simulink model "part2"  (R2025b)
settings: Solver=FixedStepAuto  StartTime=0.0  StopTime=t_end  FixedStep=h  RelTol=1e-3
values from neighbouring files (symbols this model uses):
  alpha = wind_coeff(:,1)*pi/180    [windCoefficients.m]
  Aw = [zeros(3,3), eye(3) ... (first row only)    [cal_jacobian.m]    (also in init.m = [zeros(3) eye(3))
  C_pitch = wind_coeff(:,6)    [windCoefficients.m]
  C_roll = wind_coeff(:,5)    [windCoefficients.m]
  C_yaw = wind_coeff(:,7)    [windCoefficients.m]
  Cw = [zeros(3) eye(3)]    [init.m]
  Cx = wind_coeff(:,2)    [windCoefficients.m]
  Cy = wind_coeff(:,3)    [windCoefficients.m]
  Cz = wind_coeff(:,4)    [windCoefficients.m]
  D = -[Xu  0   0 ... (first row only)    [ai_lqr.m]    (also in cal_jacobian.m = diag([d11, d22, d33]); compute_dp_gain_schedule.m = [2.6486e5       0           0; compute_integral_dp_gain_schedule.m = [2.6486e5       0           0; dp_lqSetPointTrack.m = [2.6486e5       0           0)
  K1 = [k11 0 0 ... (first row only)    [init.m]
  K2 = [k2 0 0 ... (first row only)    [init.m]
  K3 = [7.0184e6*0.1      0              0 ... (first row only)    [init.m]
  K4 = [7.0184e6*100      0              0 ... (first row only)    [init.m]
  Kp = M*Omega_n^2    [init_pid.m]
  M_inv = inv(M)    [cal_jacobian.m]    (also in init.m = M\eye(3))
  mu = 0.001    [SimulationParam.m]
  mu_w = 0.001    [init.m]
  psi_max = psi_wind_0 + deg2rad(5)    [init.m]
  psi_min = psi_wind_0 - deg2rad(5)    [init.m]
  psi_wind_0 = deg2rad(180)    [init.m]
  T_inv = T_mat\eye(3)    [init.m]
  U_bar = 10    [SimulationParam.m]    (also in init.m)
  Vc = -0.2    [SimulationParam.m]
  vessel = computeManeuveringModel(vessel, omega_p, plotFlag)    [init_pid.m]
undefined symbols (not defined in the file or in its folder): currentMode, DiscIntNeverNeededParam, Hoerner, Kd, Ki, thrusters
libraries: marine_gnc x2, marine_hydro x2, simulink x2
settings Model: Creator=jonbjor  LastModifiedBy=porpl
settings SolverCC: AlgebraicLoopSolver=TrustRegion
settings DataIOCC: ReturnWorkspaceOutputs=off
settings DebuggingCC: UnconnectedInputMsg=warning  UnconnectedOutputMsg=warning  UnconnectedLineMsg=warning  ArithmeticOperatorsInVariantConditions=warning
settings ModelReferenceCC: EnableRefExpFcnMdlSchedulingChecks=on
settings SFSimCC: SimUseLocalCustomCode=off  CustomCodeUndefinedFunction=UseInterfaceOnly
settings RTWCC: RTWUseLocalCustomCode=off  GPUComputeCapability=3.5  DLArmComputeVersion=19.05

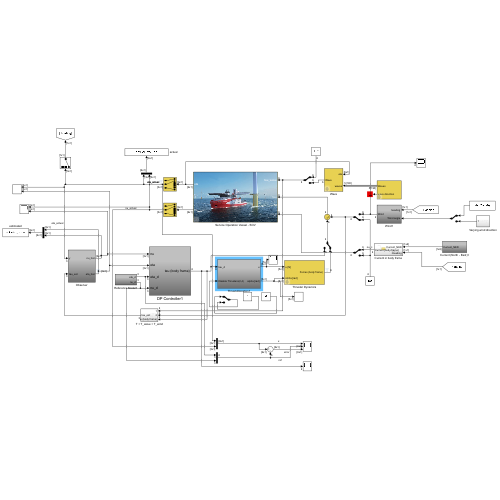
[thumbnail: Simulink's stored preview of the top-level diagram]
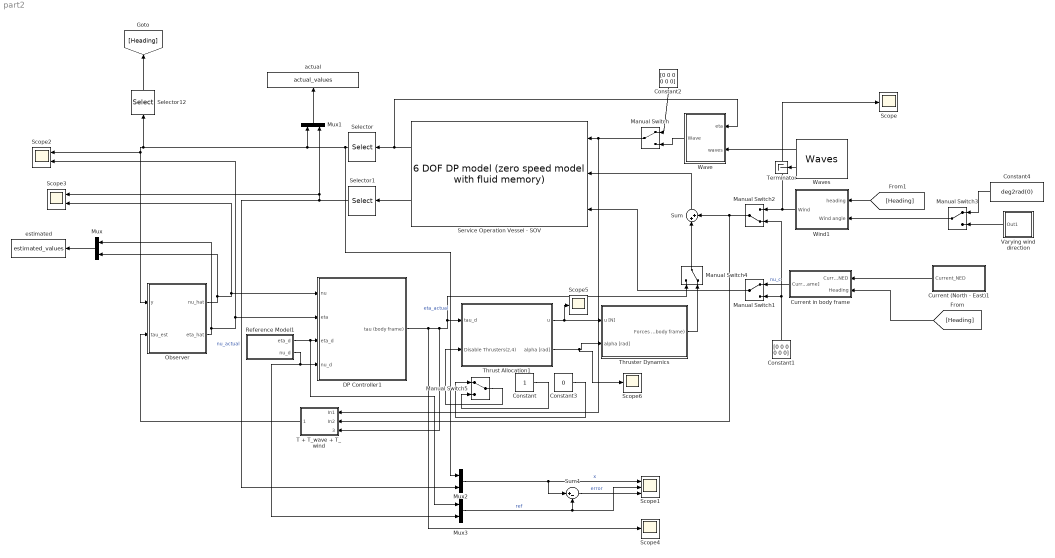
== system part2 ==
  Constant : Constant
  Constant1 : Constant  Value=[0 0 0 0 0 0]
  Constant2 : Constant  Value=[0 0 0 0 0 0]
  Constant3 : Constant  Value=0
  Constant4 : Constant  Value=deg2rad(0)
  Current (North - East)1 : Subsystem
  Current in body frame : Subsystem
  DP Controller1 : Subsystem
  Manual Switch{,1,3,5} (4 alike) : ManualSwitch
  Manual Switch2 : ManualSwitch  CurrentSetting=0
  Manual Switch4 : ManualSwitch  CurrentSetting=0
  Mux{,1..3} (4 alike) : Mux  Inputs=2
  Observer : Subsystem
  Reference Model1 : Subsystem
  Scope{,4..6} (4 alike) : Scope
      Scope settings: ActiveDisplayYMinimum=-27005.889038200934  ActiveDisplayYMaximum=47077.2958443451  DataLoggingVariableName=ScopeData3
      Scope4 settings: ActiveDisplayYMinimum=-372909.30301952863  ActiveDisplayYMaximum=43481.218565711795  DataLoggingVariableName=ScopeData2
      Scope5 settings: ActiveDisplayYMinimum=-1898.0839935154861  ActiveDisplayYMaximum=1606.2165796960817
      Scope6 settings: ActiveDisplayYMinimum=-0.21991075145912925  ActiveDisplayYMaximum=1.7697637799342327  DataLoggingVariableName=ScopeData4
  Scope1 : Scope  NumInputPorts=3
      settings: ActiveDisplayYMinimum=-69.3036258603526  ActiveDisplayYMaximum=7.7004028733725089
  Scope2 : Scope  NumInputPorts=2
      settings: ActiveDisplayYMinimum=-9.7951804135394376  ActiveDisplayYMaximum=18.071809579069871  DataLoggingVariableName=ScopeData5
  Scope3 : Scope  NumInputPorts=2
      settings: ActiveDisplayYMinimum=-1.3881269624266319  ActiveDisplayYMaximum=2.4884875921743972  DataLoggingVariableName=ScopeData6
  Selector : Selector  InputPortWidth=6  IndexOptions=Index vector (dialog)  Indices=[1 2 6]  OutputSizes=1
  Selector1 : Selector  InputPortWidth=6  IndexOptions=Index vector (dialog)  Indices=[1 2 6]  OutputSizes=1
  Selector12 : Selector  InputPortWidth=3  IndexOptions=Index vector (dialog)  Indices=[ 3]  OutputSizes=1
  Service Operation Vessel - SOV : marine_hydro/Hydro Library/6 DOF DP model  (zero speed model with fluid memory)  ABC=vesselABC  rho=1025  Axc=0.9*vessel.main.T*vessel.main.B  Ayc=0.9*vessel.main.T*vessel.main.Lpp  CX=1  CY_2D=Hoerner(vessel.main.B,vessel.main.T)  Bv=vessel.Bv  mask(6 DOF zero speed model){}
      link override "Integrator1 ": InitialCondition=nu0
      link override Integrator2: InitialCondition=eta0
      settings: SourceProductName=MSS Hydro
      mask Display:
      | image('SOV.jpg');
      | color('white'); port_label('output', 1, 'eta')
      | color('white'); port_label('output', 2, 'nu')
      | color('white'); port_label('input', 1, 'tau_wave')
      | color('white'); port_label('input', 2, 'tau')
      | color('white'); port_label('input', 3, 'nu_c')
  Sum : Sum  Inputs=|++
  Sum1 : Sum  Inputs=|+-
  T + T_wave + T_wind : Subsystem
  Terminator : Terminator
  Thrust Allocation1 : Subsystem
  Thruster Dynamics : Subsystem  mask{thrusterfault=off}
      mask prompts: thrusterfault "Fault on thruster #2 and #4?"
  Varying wind direction : Subsystem
  Wave : Subsystem  mask{waveforces=on}
      mask prompts: waveforces "Waveforces enabled"
  Waves : marine_gnc/Environment/Waves/Waves  spectrum_type=ITTC  disp_flag=on  plot_spectrum=off  plot_realization=off  hs=5  omega_peak=pi/10  psi_mean=0  gamma=-1  spread=2  depth=inf  nfreq=20  ndir=10  energylim=0.005  freq_cutoff=3  dir_cutoff=0  rand_seed=123  rand_freq=on  rand_dir=on  Zeta_a=0  Omega=0  Phase=0  Wavenum=0  Psi=0
      settings: SourceProductName=MSS GNC
  Wind1 : Subsystem
  actual : ToWorkspace  VariableName=actual_values  SampleTime=-1
  estimated : ToWorkspace  VariableName=estimated_values  SampleTime=-1
  wires:
  Service Operation Vessel - SOV/2 -> Selector1/1
  DP Controller1/1(tau (body frame)) -> Scope4/1, Thrust Allocation1/1(tau_d), Manual Switch4/1, T + T_wave + T_wind/3(tau (body frame))
  Service Operation Vessel - SOV/1 -> Wave/1(eta), Selector/1
  Waves/1 -> Wave/2(waves)
  Waves/2 -> Terminator/1
  Sum/1 -> Service Operation Vessel - SOV/2
  Selector/1 -> Mux2/1, Observer/1(y), Scope2/1, Selector12/1, Mux1/1  "eta_actual"
  Current (North - East)1/1(Current_NED) -> Current in body frame/1(Current_NED)
  Current in body frame/1(Current [body-frame]) -> Manual Switch1/1  "nu_c"
  Manual Switch1/1 -> Service Operation Vessel - SOV/3
  Constant1/1 -> Manual Switch2/2, Manual Switch1/2
  Wind1/1(Wind) -> Scope/1, Manual Switch2/1
  Manual Switch2/1 -> T + T_wave + T_wind/2(In2), Sum/2
  Observer/1(nu_hat) -> Scope3/2, DP Controller1/1(nu), Mux/2
  Observer/2(eta_hat) -> Scope2/2, DP Controller1/2(eta), Mux/1
  Selector1/1 -> Mux2/2, Mux1/2, Scope3/1  "nu_actual"
  Wave/1(Wave) -> Manual Switch/2
  Mux/1 -> estimated/1
  Mux1/1 -> actual/1
  Selector12/1 -> [Heading]
  [Heading] -> Current in body frame/2(Heading)
  [Heading] -> Wind1/1(heading)
  Constant4/1 -> Manual Switch3/1
  Manual Switch3/1 -> Wind1/2(Wind angle)
  Varying wind direction/1(Out1) -> Manual Switch3/2
  T + T_wave + T_wind/1(tau_est) -> Observer/2(tau_est)
  Thruster Dynamics/1("Forces (body frame) ") -> Manual Switch4/2
  Manual Switch4/1 -> Sum/1
  Mux2/1 -> Sum1/1, Scope1/1  "x"
  Sum1/1 -> Scope1/3  "error"
  Manual Switch/1 -> T + T_wave + T_wind/1(In1), Service Operation Vessel - SOV/1
  Constant2/1 -> Manual Switch/1
  Reference Model1/1(eta_d) -> Mux3/1, DP Controller1/3(eta_d)
  Reference Model1/2(nu_d) -> DP Controller1/4(nu_d), Mux3/2
  Mux3/1 -> Scope1/2, Sum1/2  "ref"
  Constant/1 -> Manual Switch5/2
  Manual Switch5/1 -> Thrust Allocation1/2(Disable Thrusters(2,4))
  Thrust Allocation1/1(u) -> Scope5/1, Thruster Dynamics/1(u [N])
  Thrust Allocation1/2(alpha [rad]) -> Scope6/1, Thruster Dynamics/2(alpha [rad])
  Constant3/1 -> Manual Switch5/1

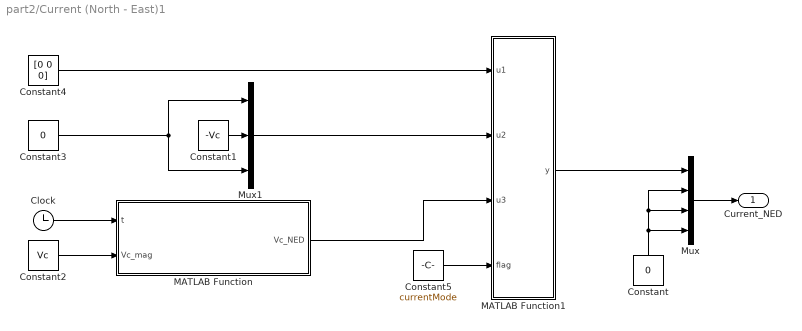
== system part2/Current (North - East)1 ==
  Clock : Clock
  Constant : Constant  Value=0
  Constant1 : Constant  Value=-Vc
  Constant2 : Constant  Value=Vc
  Constant3 : Constant  Value=0
  Constant4 : Constant  Value=[0 0 0]
  Constant5 : Constant  Value=currentMode
  MATLAB Function : MATLAB Function  TreatAsAtomicUnit=on
  MATLAB Function1 : MATLAB Function  TreatAsAtomicUnit=on
  Mux : Mux
  Mux1 : Mux  Inputs=3
  Current_NED : Outport  VectorParamsAs1DForOutWhenUnconnected=off
  wires:
  Constant1/1 -> Mux1/2
  Constant3/1 -> Mux1/1, Mux1/3
  Clock/1 -> MATLAB Function/1(t)
  Constant2/1 -> MATLAB Function/2(Vc_mag)
  Mux/1 -> Current_NED/1
  Constant/1 -> Mux/2, Mux/3, Mux/4
  Mux1/1 -> MATLAB Function1/2(u2)
  MATLAB Function/1(Vc_NED) -> MATLAB Function1/3(u3)
  Constant4/1 -> MATLAB Function1/1(u1)
  Constant5/1 -> MATLAB Function1/4(flag)
  MATLAB Function1/1(y) -> Mux/1

== system part2/Current in body frame ==
  Current_NED : Inport
  Heading : Inport  Port=2
  Constant : Constant  Value=0
  Mux : Mux
  Transposed rotation matrix in yaw : marine_gnc/Models/ Kinematics/Transposed rotation  matrix in yaw
      settings: SourceProductName=MSS GNC
  Current [body-frame] : Outport
  wires:
  Current_NED/1 -> Transposed rotation matrix in yaw/2
  Transposed rotation matrix in yaw/1 -> Mux/1
  Heading/1 -> Transposed rotation matrix in yaw/1
  Mux/1 -> Current [body-frame]/1
  Constant/1 -> Mux/4, Mux/3, Mux/2

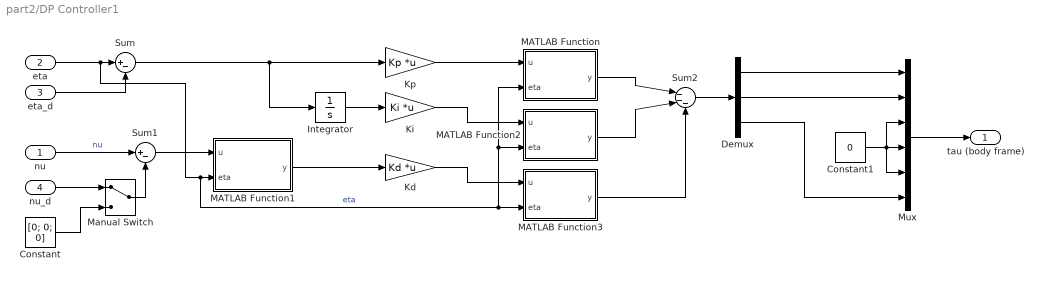
== system part2/DP Controller1 ==
  nu : Inport
  eta : Inport  Port=2
  eta_d : Inport  Port=3
  nu_d : Inport  Port=4
  Constant : Constant  Value=[0; 0; 0]
  Constant1 : Constant  Value=0
  Demux : Demux  Outputs=3
  Integrator : Integrator
  Kd : Gain  Gain=Kd  Multiplication=Matrix(K*u)
  Ki : Gain  Gain=Ki  Multiplication=Matrix(K*u)
  Kp : Gain  Gain=Kp  Multiplication=Matrix(K*u)
  MATLAB Function : MATLAB Function  TreatAsAtomicUnit=on
  MATLAB Function1 : MATLAB Function  TreatAsAtomicUnit=on
  MATLAB Function2 : MATLAB Function  TreatAsAtomicUnit=on
  MATLAB Function3 : MATLAB Function  TreatAsAtomicUnit=on
  Manual Switch : ManualSwitch
  Mux : Mux  Inputs=6
  Sum : Sum  Inputs=|+-
  Sum1 : Sum  Inputs=|+-
  Sum2 : Sum  Inputs=|---
  tau (body frame) : Outport  VectorParamsAs1DForOutWhenUnconnected=off
  wires:
  Demux/1 -> Mux/1
  Demux/2 -> Mux/2
  Demux/3 -> Mux/6
  Constant1/1 -> Mux/5, Mux/3, Mux/4
  Mux/1 -> tau (body frame)/1
  eta/1 -> MATLAB Function3/2(eta), MATLAB Function/2(eta), MATLAB Function2/2(eta), MATLAB Function1/2(eta), Sum/1  "eta"
  eta_d/1 -> Sum/2
  nu/1 -> Sum1/1  "nu"
  nu_d/1 -> Manual Switch/1
  Manual Switch/1 -> Sum1/2
  Constant/1 -> Manual Switch/2
  Sum1/1 -> MATLAB Function1/1(u)
  Sum/1 -> Integrator/1, Kp/1
  Integrator/1 -> Ki/1
  MATLAB Function1/1(y) -> Kd/1
  Kp/1 -> MATLAB Function/1(u)
  Ki/1 -> MATLAB Function2/1(u)
  Kd/1 -> MATLAB Function3/1(u)
  Sum2/1 -> Demux/1
  MATLAB Function/1(y) -> Sum2/1
  MATLAB Function2/1(y) -> Sum2/2
  MATLAB Function3/1(y) -> Sum2/3

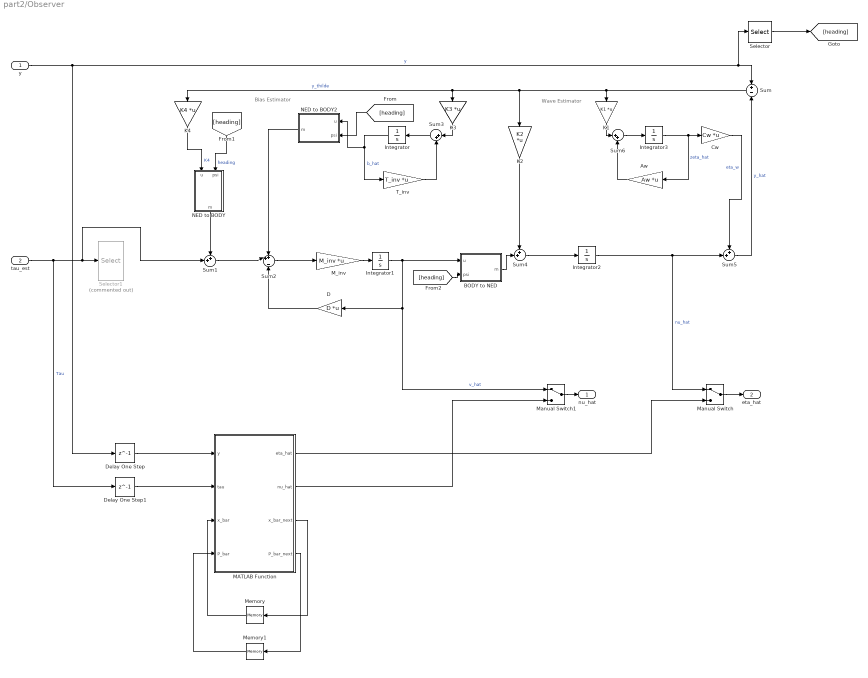
== system part2/Observer ==
  note: Wave Estimator
  note: Bias Estimator
  y : Inport
  tau_est : Inport  Port=2
  Aw : Gain  Gain=Aw  Multiplication=Matrix(K*u)
  BODY to NED : MATLAB Function  TreatAsAtomicUnit=on
  Cw : Gain  Gain=Cw  Multiplication=Matrix(K*u)
  D : Gain  Gain=D  Multiplication=Matrix(K*u)
  Delay One Step : Delay  DelayLength=1
  Delay One Step1 : Delay  DelayLength=1
  Integrator{,1..3} (4 alike) : Integrator
  K1 : Gain  Gain=K1  Multiplication=Matrix(K*u)
  K2 : Gain  Gain=K2  Multiplication=Matrix(K*u)
  K3 : Gain  Gain=K3  Multiplication=Matrix(K*u)
  K4 : Gain  Gain=K4  Multiplication=Matrix(K*u)
  MATLAB Function : MATLAB Function  TreatAsAtomicUnit=on
  M_inv : Gain  Gain=M_inv  Multiplication=Matrix(K*u)
  Manual Switch : ManualSwitch
  Manual Switch1 : ManualSwitch
  Memory : Memory
  Memory1 : Memory
  NED to BODY : MATLAB Function  TreatAsAtomicUnit=on
  NED to BODY2 : MATLAB Function  TreatAsAtomicUnit=on
  Selector : Selector  InputPortWidth=3  IndexOptions=Index vector (dialog)  Indices=[3]  OutputSizes=1
  Selector1 : Selector  Commented=on  InputPortWidth=6  IndexOptions=Index vector (dialog)  Indices=[1 2 6]  OutputSizes=1
  Sum : Sum  Inputs=+|-
  Sum1 : Sum  Inputs=++|
  Sum2 : Sum  Inputs=++|-
  Sum3 : Sum  Inputs=|++
  Sum4 : Sum  Inputs=++|
  Sum5 : Sum  Inputs=++|
  Sum6 : Sum  Inputs=|++
  T_inv : Gain  Gain=T_inv  Multiplication=Matrix(K*u)
  nu_hat : Outport  VectorParamsAs1DForOutWhenUnconnected=off
  eta_hat : Outport  Port=2  VectorParamsAs1DForOutWhenUnconnected=off
  wires:
  y/1 -> Delay One Step/1, Selector/1, Sum/1  "y"
  Sum5/1 -> Sum/2  "y_hat"
  Sum/1 -> K4/1, K3/1, K2/1, K1/1  "y_thilde"
  NED to BODY/1(m) -> Sum1/1
  Sum1/1 -> Sum2/2
  Integrator/1 -> NED to BODY2/1(u), T_inv/1  "b_hat"
  NED to BODY2/1(m) -> Sum2/1
  T_inv/1 -> Sum3/2
  K3/1 -> Sum3/1
  Sum3/1 -> Integrator/1
  Sum2/1 -> M_inv/1
  M_inv/1 -> Integrator1/1
  Integrator1/1 -> BODY to NED/1(u), Manual Switch1/1, D/1  "v_hat"
  D/1 -> Sum2/3
  K2/1 -> Sum4/1
  Sum4/1 -> Integrator2/1
  Integrator2/1 -> Manual Switch/1, Sum5/2  "nu_hat"
  Integrator3/1 -> Aw/1, Cw/1  "zeta_hat"
  K1/1 -> Sum6/1
  Sum6/1 -> Integrator3/1
  Aw/1 -> Sum6/2
  Cw/1 -> Sum5/1  "eta_w"
  Selector/1 -> [heading]
  [heading] -> BODY to NED/2(psi)
  tau_est/1 -> Delay One Step1/1, Sum1/2, Selector1/1  "Tau"
  [heading] -> NED to BODY/2(psi)  "heading"
  K4/1 -> NED to BODY/1(u)  "K4"
  [heading] -> NED to BODY2/2(psi)
  BODY to NED/1(m) -> Sum4/2
  Manual Switch/1 -> eta_hat/1
  Manual Switch1/1 -> nu_hat/1
  MATLAB Function/2(nu_hat) -> Manual Switch1/2
  MATLAB Function/1(eta_hat) -> Manual Switch/2
  Delay One Step/1 -> MATLAB Function/1(y)
  Delay One Step1/1 -> MATLAB Function/2(tau)
  MATLAB Function/3(x_bar_next) -> Memory/1
  MATLAB Function/4(P_bar_next) -> Memory1/1
  Memory/1 -> MATLAB Function/3(x_bar)
  Memory1/1 -> MATLAB Function/4(P_bar)

== system part2/Reference Model1 ==
  Demux : Demux  Outputs=6
  From Workspace1 : FromWorkspace  VariableName=simin
  Mux : Mux  Inputs=3
  Mux1 : Mux  Inputs=3
  eta_d : Outport  VectorParamsAs1DForOutWhenUnconnected=off
  nu_d : Outport  Port=2
  wires:
  From Workspace1/1 -> Demux/1
  Demux/1 -> Mux/1
  Demux/2 -> Mux/2
  Demux/3 -> Mux/3
  Demux/4 -> Mux1/1
  Demux/5 -> Mux1/2
  Demux/6 -> Mux1/3
  Mux/1 -> eta_d/1
  Mux1/1 -> nu_d/1

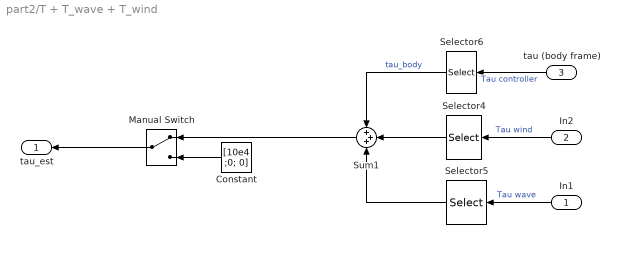
== system part2/T + T_wave + T_wind ==
  In1 : Inport
  In2 : Inport  Port=2
  tau (body frame) : Inport  Port=3
  Constant : Constant  Value=[10e4 ;0; 0]
  Manual Switch : ManualSwitch
  Selector4 : Selector  InputPortWidth=6  IndexOptions=Index vector (dialog)  Indices=[1 2 6]  OutputSizes=1
  Selector5 : Selector  InputPortWidth=6  IndexOptions=Index vector (dialog)  Indices=[1 2 6]  OutputSizes=1
  Selector6 : Selector  InputPortWidth=6  IndexOptions=Index vector (dialog)  Indices=[1 2 6]  OutputSizes=1
  Sum1 : Sum  Inputs=+++
  tau_est : Outport
  wires:
  Selector6/1 -> Sum1/1  "tau_body"
  Selector5/1 -> Sum1/3
  Constant/1 -> Manual Switch/2
  Selector4/1 -> Sum1/2
  Sum1/1 -> Manual Switch/1
  In1/1 -> Selector5/1  "Tau wave"
  In2/1 -> Selector4/1  "Tau wind"
  Manual Switch/1 -> tau_est/1
  tau (body frame)/1 -> Selector6/1  "Tau controller"

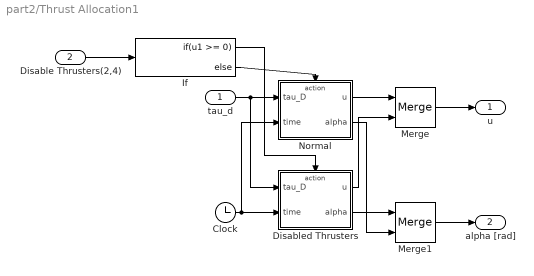
== system part2/Thrust Allocation1 ==
  tau_d : Inport  PortDimensions=6
  Disable Thrusters(2,4) : Inport  Port=2
  Clock : Clock
  Disabled Thrusters : Subsystem  TreatAsAtomicUnit=on
  If : If  IfExpression=u1 >= 0
  Merge : Merge
  Merge1 : Merge
  Normal : Subsystem  TreatAsAtomicUnit=on
  u : Outport  VectorParamsAs1DForOutWhenUnconnected=off
  alpha [rad] : Outport  Port=2  VectorParamsAs1DForOutWhenUnconnected=off
  wires:
  If/1 -> Disabled Thrusters/Action
  If/2 -> Normal/Action
  Disabled Thrusters/1(u) -> Merge/2
  tau_d/1 -> Disabled Thrusters/1(tau_D), Normal/1(tau_D)
  Clock/1 -> Normal/2(time), Disabled Thrusters/2(time)
  Normal/2(alpha) -> Merge1/2
  Normal/1(u) -> Merge/1
  Disabled Thrusters/2(alpha) -> Merge1/1
  Merge/1 -> u/1
  Merge1/1 -> alpha [rad]/1
  Disable Thrusters(2,4)/1 -> If/1

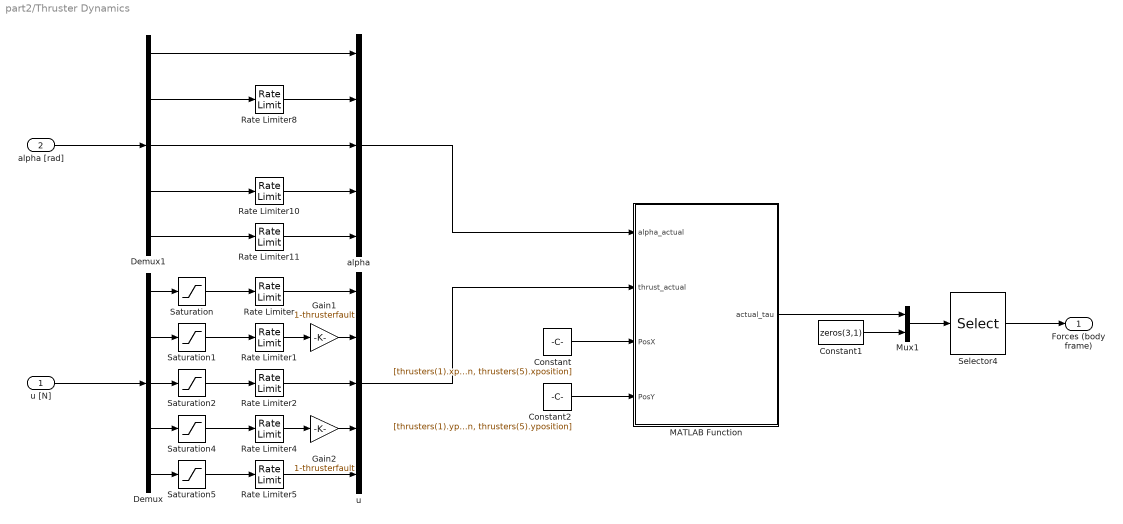
== system part2/Thruster Dynamics ==
  u [N] : Inport
  alpha [rad] : Inport  Port=2
  Constant : Constant  Value=[thrusters(1).xposition, thrusters(2).xposition, thrusters(3).xposition, thrusters(4).xposition, thrusters(5).xposition]
  Constant1 : Constant  Value=zeros(3,1)
  Constant2 : Constant  Value=[thrusters(1).yposition, thrusters(2).yposition, thrusters(3).yposition, thrusters(4).yposition, thrusters(5).yposition]
  Demux : Demux  Outputs=5
  Demux1 : Demux  Outputs=5
  Gain1 : Gain  Gain=1-thrusterfault
  Gain2 : Gain  Gain=1-thrusterfault
  MATLAB Function : MATLAB Function  TreatAsAtomicUnit=on
  Mux1 : Mux  Inputs=2
  Rate Limiter : RateLimiter  RisingSlewLimit=thrusters(1).rate  FallingSlewLimit=-thrusters(1).rate  SampleTimeMode=inherited
  Rate Limiter1 : RateLimiter  RisingSlewLimit=thrusters(2).rate  FallingSlewLimit=-thrusters(2).rate  SampleTimeMode=inherited
  Rate Limiter10 : RateLimiter  RisingSlewLimit=thrusters(4).rotationspeed  FallingSlewLimit=-thrusters(4).rotationspeed  SampleTimeMode=inherited
  Rate Limiter11 : RateLimiter  RisingSlewLimit=thrusters(5).rotationspeed  FallingSlewLimit=-thrusters(5).rotationspeed  SampleTimeMode=inherited
  Rate Limiter2 : RateLimiter  RisingSlewLimit=thrusters(3).rate  FallingSlewLimit=-thrusters(3).rate  SampleTimeMode=inherited
  Rate Limiter4 : RateLimiter  RisingSlewLimit=thrusters(4).rate  FallingSlewLimit=-thrusters(4).rate  SampleTimeMode=inherited
  Rate Limiter5 : RateLimiter  RisingSlewLimit=thrusters(5).rate  FallingSlewLimit=-thrusters(5).rate  SampleTimeMode=inherited
  Rate Limiter8 : RateLimiter  RisingSlewLimit=thrusters(2).rotationspeed  FallingSlewLimit=-thrusters(2).rotationspeed  SampleTimeMode=inherited
  Saturation : Saturate  UpperLimit=thrusters(1).thrust  LowerLimit=-thrusters(1).thrust
  Saturation1 : Saturate  UpperLimit=thrusters(2).thrust  LowerLimit=-thrusters(2).thrust
  Saturation2 : Saturate  UpperLimit=thrusters(3).thrust  LowerLimit=-thrusters(3).thrust
  Saturation4 : Saturate  UpperLimit=thrusters(4).thrust  LowerLimit=-thrusters(4).thrust
  Saturation5 : Saturate  UpperLimit=thrusters(5).thrust  LowerLimit=-thrusters(5).thrust
  Selector4 : Selector  InputPortWidth=6  IndexOptions=Index vector (dialog)  Indices=[1 2 4 5 6 3]  OutputSizes=1
  alpha : Mux  Inputs=5
  u : Mux  Inputs=5
  "Forces (body frame) " : Outport  VectorParamsAs1DForOutWhenUnconnected=off
  wires:
  Rate Limiter2/1 -> u/3
  Saturation/1 -> Rate Limiter/1
  Mux1/1 -> Selector4/1
  Constant1/1 -> Mux1/2
  Saturation4/1 -> Rate Limiter4/1
  Demux/2 -> Saturation1/1
  Saturation1/1 -> Rate Limiter1/1
  Demux/1 -> Saturation/1
  Demux/3 -> Saturation2/1
  Saturation2/1 -> Rate Limiter2/1
  Selector4/1 -> "Forces (body frame) "/1
  Gain1/1 -> u/2
  Rate Limiter1/1 -> Gain1/1
  Rate Limiter/1 -> u/1
  Rate Limiter4/1 -> Gain2/1
  Saturation5/1 -> Rate Limiter5/1
  u [N]/1 -> Demux/1
  alpha [rad]/1 -> Demux1/1
  Constant/1 -> MATLAB Function/3(PosX)
  Constant2/1 -> MATLAB Function/4(PosY)
  u/1 -> MATLAB Function/2(thrust_actual)
  alpha/1 -> MATLAB Function/1(alpha_actual)
  MATLAB Function/1(actual_tau) -> Mux1/1
  Rate Limiter10/1 -> alpha/4
  Demux1/4 -> Rate Limiter10/1
  Demux1/5 -> Rate Limiter11/1
  Rate Limiter11/1 -> alpha/5
  Demux1/1 -> alpha/1
  Gain2/1 -> u/4
  Demux/4 -> Saturation4/1
  Demux/5 -> Saturation5/1
  Rate Limiter5/1 -> u/5
  Demux1/2 -> Rate Limiter8/1
  Rate Limiter8/1 -> alpha/2
  Demux1/3 -> alpha/3

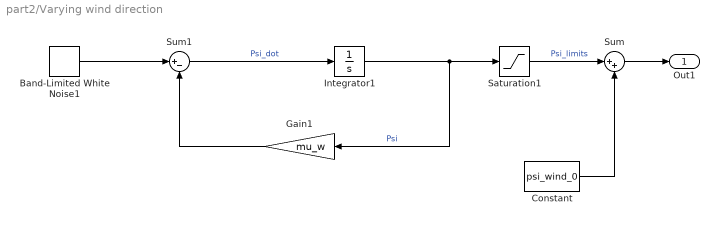
== system part2/Varying wind direction ==
  Band-Limited White Noise1 : simulink/Sources/Band-Limited White Noise  Cov=0.00005  Ts=0.1  seed=[23381]
  Constant : Constant  Value=psi_wind_0
  Gain1 : Gain  Gain=mu_w
  Integrator1 : Integrator
  Saturation1 : Saturate  UpperLimit=psi_max  LowerLimit=psi_min
  Sum : Sum  Inputs=|++
  Sum1 : Sum  Inputs=|+-
  Out1 : Outport
  wires:
  Gain1/1 -> Sum1/2
  Constant/1 -> Sum/2
  Sum/1 -> Out1/1
  Sum1/1 -> Integrator1/1  "Psi_dot"
  Band-Limited White Noise1/1 -> Sum1/1
  Integrator1/1 -> Gain1/1, Saturation1/1  "Psi"
  Saturation1/1 -> Sum/1  "Psi_limits"

== system part2/Wave ==
  eta : Inport
  waves : Inport  Port=2
  Gain : Gain  Gain=waveforces
  Sum : Sum
  Wave loads (U=0) : marine_hydro/Hydro Library/Wave loads (U=0)  SystemSampleTime=-1  VariantActivationTime=update diagram  EmptyChoice=off  PassThrough=off  PassThroughVariantControl=(default)  EmptyChoiceVariantControl=(default)  AllowFlexibleInterface=on  Latency=0  AutoFrameSizeCalculation=off
      settings: SourceProductName=MSS Hydro
  Wave : Outport  VectorParamsAs1DForOutWhenUnconnected=off
  wires:
  eta/1 -> Wave loads (U=0)/1
  waves/1 -> Wave loads (U=0)/2
  Sum/1 -> Gain/1
  Wave loads (U=0)/1 -> Sum/1
  Wave loads (U=0)/2 -> Sum/2
  Gain/1 -> Wave/1

== system part2/Wind1 ==
  heading : Inport
  Wind angle : Inport  Port=2
  Subsystem : Subsystem
  Sum : Sum  Inputs=|+-
  Wind Speed : Subsystem
  Wind : Outport  VectorParamsAs1DForOutWhenUnconnected=off
  wires:
  Wind Speed/1(Out1) -> Subsystem/2(Vw)
  Wind angle/1 -> Sum/1
  heading/1 -> Sum/2
  Sum/1 -> Subsystem/1(alpha_r)
  Subsystem/1(Wind) -> Wind/1

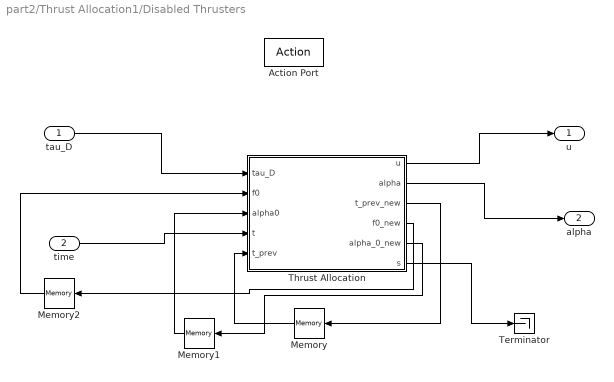
== system part2/Thrust Allocation1/Disabled Thrusters ==
  tau_D : Inport
  time : Inport  Port=2
  Action Port : ActionPort  ActionPortLabel=if(u1 >= 0)
  Memory : Memory
  Memory1 : Memory  InitialCondition=[pi/2; 0; pi/2; 0; 0]
  Memory2 : Memory  InitialCondition=[0; 0; 0; 0; 0]
  Terminator : Terminator
  Thrust Allocation : MATLAB Function  TreatAsAtomicUnit=on
  u : Outport
  alpha : Outport  Port=2
  wires:
  time/1 -> Thrust Allocation/4(t)
  Thrust Allocation/2(alpha) -> alpha/1
  Thrust Allocation/1(u) -> u/1
  tau_D/1 -> Thrust Allocation/1(tau_D)
  Thrust Allocation/6(s) -> Terminator/1
  Memory/1 -> Thrust Allocation/5(t_prev)
  Thrust Allocation/3(t_prev_new) -> Memory/1
  Memory1/1 -> Thrust Allocation/3(alpha0)
  Thrust Allocation/5(alpha_0_new) -> Memory1/1
  Thrust Allocation/4(f0_new) -> Memory2/1
  Memory2/1 -> Thrust Allocation/2(f0)

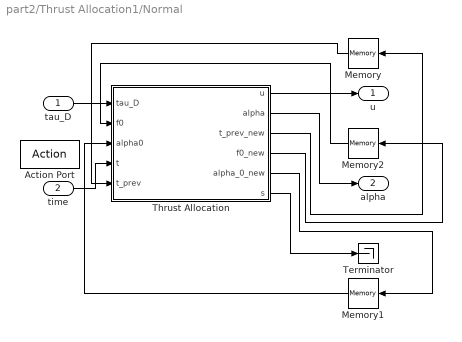
== system part2/Thrust Allocation1/Normal ==
  tau_D : Inport
  time : Inport  Port=2
  Action Port : ActionPort  ActionPortLabel=else
  Memory : Memory
  Memory1 : Memory  InitialCondition=[pi/2; 0; pi/2; 0; 0]
  Memory2 : Memory  InitialCondition=[0; 0; 0; 0; 0]
  Terminator : Terminator
  Thrust Allocation : MATLAB Function  TreatAsAtomicUnit=on
  u : Outport
  alpha : Outport  Port=2
  wires:
  Memory1/1 -> Thrust Allocation/3(alpha0)
  Thrust Allocation/5(alpha_0_new) -> Memory1/1
  Thrust Allocation/3(t_prev_new) -> Memory/1
  Thrust Allocation/1(u) -> u/1
  time/1 -> Thrust Allocation/4(t)
  tau_D/1 -> Thrust Allocation/1(tau_D)
  Thrust Allocation/6(s) -> Terminator/1
  Thrust Allocation/4(f0_new) -> Memory2/1
  Thrust Allocation/2(alpha) -> alpha/1
  Memory/1 -> Thrust Allocation/5(t_prev)
  Memory2/1 -> Thrust Allocation/2(f0)

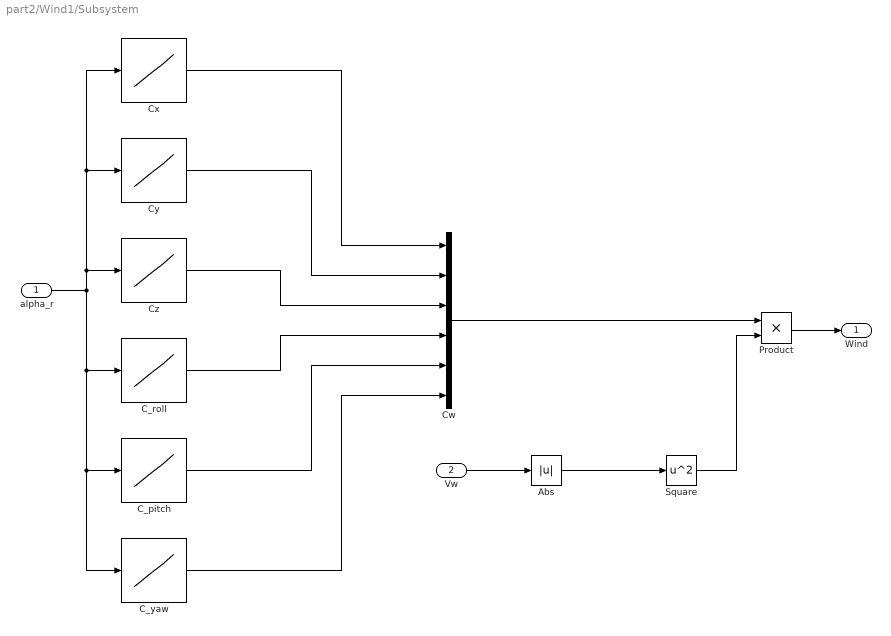
== system part2/Wind1/Subsystem ==
  alpha_r : Inport
  Vw : Inport  Port=2
  Abs : Abs  SaturateOnIntegerOverflow=off
  C_pitch : Lookup_n-D  NumberOfTableDimensions=1  BreakpointsForDimension1=alpha  Table=C_pitch  InternalRulePriority=Speed  RndMeth=Simplest
  C_roll : Lookup_n-D  NumberOfTableDimensions=1  BreakpointsForDimension1=alpha  Table=C_roll  InternalRulePriority=Speed  RndMeth=Simplest
  C_yaw : Lookup_n-D  NumberOfTableDimensions=1  BreakpointsForDimension1=alpha  Table=C_yaw  InternalRulePriority=Speed  RndMeth=Simplest
  Cw : Mux  Inputs=6
  Cx : Lookup_n-D  NumberOfTableDimensions=1  BreakpointsForDimension1=alpha  Table=Cx  InternalRulePriority=Speed  RndMeth=Simplest
  Cy : Lookup_n-D  NumberOfTableDimensions=1  BreakpointsForDimension1=alpha  Table=Cy  InternalRulePriority=Speed  RndMeth=Simplest
  Cz : Lookup_n-D  NumberOfTableDimensions=1  BreakpointsForDimension1=alpha  Table=Cz  InternalRulePriority=Speed  RndMeth=Simplest
  Product : Product
  Square : Math  Operator=square
  Wind : Outport  VectorParamsAs1DForOutWhenUnconnected=off
  wires:
  Vw/1 -> Abs/1
  Cy/1 -> Cw/2
  C_roll/1 -> Cw/4
  Cw/1 -> Product/1
  C_pitch/1 -> Cw/5
  Square/1 -> Product/2
  alpha_r/1 -> C_yaw/1, C_pitch/1, C_roll/1, Cx/1, Cy/1, Cz/1
  Cz/1 -> Cw/3
  C_yaw/1 -> Cw/6
  Cx/1 -> Cw/1
  Abs/1 -> Square/1
  Product/1 -> Wind/1

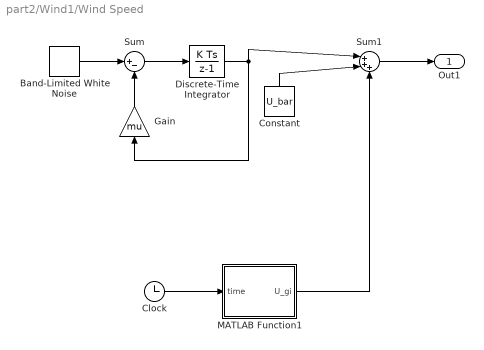
== system part2/Wind1/Wind Speed ==
  Band-Limited White Noise : simulink/Sources/Band-Limited White Noise  Cov=power_w_c  Ts=0.1  seed=[23341]
  Clock : Clock
  Constant : Constant  Value=U_bar
  Discrete-Time Integrator : DiscreteIntegrator  SampleTime=-1  ICPrevOutput=DiscIntNeverNeededParam  ICPrevScaledInput=DiscIntNeverNeededParam
  Gain : Gain  Gain=mu
  MATLAB Function1 : MATLAB Function  TreatAsAtomicUnit=on  SystemSampleTime=0.1
  Sum : Sum  Inputs=|+-
  Sum1 : Sum  Inputs=|+++
  Out1 : Outport
  wires:
  Discrete-Time Integrator/1 -> Gain/1, Sum1/1
  Gain/1 -> Sum/2
  Constant/1 -> Sum1/2
  Sum/1 -> Discrete-Time Integrator/1
  Band-Limited White Noise/1 -> Sum/1
  Sum1/1 -> Out1/1
  Clock/1 -> MATLAB Function1/1(time)
  MATLAB Function1/1(U_gi) -> Sum1/3

== matlab function part2/DP Controller1/MATLAB Function2 ==
  data: u input; y output; eta input
function y = Rz_psi_T(u, eta)
y = zeros(3,1);

psi = eta(3);

c = cos(psi); s = sin(psi);

R = [c -s  0;
     s  c  0;
     0  0  1];

y = R'*u;

== matlab function part2/DP Controller1/MATLAB Function3 ==
  data: u input; y output; eta input
function y = Rz_psi_T(u, eta)
y = zeros(3,1);

psi = eta(3);

c = cos(psi); s = sin(psi);

R = [c -s  0;
     s  c  0;
     0  0  1];

y = R'*u;

== matlab function part2/Observer/MATLAB Function ==
  data: y input; eta_hat output; tau input; x_bar input; P_bar input; nu_hat output; x_bar_next output; P_bar_next output
function [eta_hat, nu_hat, x_bar_next, P_bar_next] = ekf(y, tau, x_bar, P_bar)
% This function implements a 15-state EKF for one time step.
%
% State Vector Order: x = [epsi, eta, b, nu]' (15x1)
%   epsi: [epsi1, epsi2, epsi3, epsi4, epsi5, epsi6]' (1-6)
%   eta: [x, y, psi]' (7-9)
%   b: [bx, by, bpsi]' (10-12)
%   nu: [u, v, r]' (13-15)
%
% Input Arguments:
%   y      - Measurement vector [x, y, psi]' (3x1)
%   tau    - Control force vector [tau_x, tau_y, tau_psi]' (3x1)
%   x_bar  - Previous State Estimate x_hat[k|k] (15x1)
%   P_bar  - Previous Covariance Matrix P[k|k] (15x15)
%
% Output Arguments:
%   eta_hat     - Estimated position/heading [x, y, psi]' (3x1)
%   nu_hat      - Estimated body-fixed velocity [u, v, r]' (3x1)
%   x_bar_next  - Updated state estimate x_hat[k+1|k+1] (15x1)
%   P_bar_next  - Updated covariance matrix P[k+1|k+1] (15x15)

    persistent Ts M D G A_w C_w Q R I I_15
    persistent m11 m22 m33 d11 d22 d33 Tb1 Tb2 Tb3
    persistent omega1 omega2 omega3 zeta1 zeta2 zeta3
    
    if isempty(M)
        % Sampling time 
        Ts = 0.1; 
        
        % Vessel Mass Matrix (Diagonal elements)
        M = [7.0184e6      0              0;
             0        8.5464e6   -4.4678e7;
             0       -4.5028e5    4.0504e9];
        
        m11 = M(1,1);
        m22 = M(2,2);
        m33 = M(3,3);
        
        % Damping matrix (Diagonal elements)
        D = [2.6486e5     0           0;
             0        8.8164e5       0;
             0             0     3.3774e8];
        
        d11 = D(1,1);
        d22 = D(2,2);
        d33 = D(3,3);
        
        G = zeros(3, 3);   % Restoring forces
        I = eye(3);
        I_15 = eye(15);
        
        % Wave Model Parameters
        omega1 = pi/10; 
        omega2 = pi/10;
        omega3 = pi/10;
        zeta1 = 0.1;
        zeta2 = 0.1;
        zeta3 = 0.1;
        
        omega = diag([omega1, omega2, omega3]);
        gam = diag([zeta1, zeta2, zeta3]);
        
        % A_w (6x6) - Wave dynamics system matrix
        A_w = [zeros(3), I; -omega*omega, -2 * gam * omega];
        
        % C_w (3x6) - Measurement Matrix
        C_w = [I, zeros(3)]; 
        
        % Bias time constants
        Tb1 = 1000;  % Large value for slow-varying bias
        Tb2 = 1000;
        Tb3 = 1000;
        
        % Noise Covariance Matrices (Tuning Parameters) 
        Q = zeros(15, 15);
        Q(1:6, 1:6) = 1e-5 * eye(6);    % Wave (epsi)
        Q(7:9, 7:9) = 1e-4 * I;         % Position (eta)
        Q(10:12, 10:12) = 1e-6 * I;     % Bias (b)
        Q(13:15, 13:15) = 1e-4 * I;     % Velocity (nu)
        
        R = diag([0.001^2, 0.001^2, (deg2rad(0.2))^2]); % Measurement Noise
    end
    
    % Initialize on first call
    if all(x_bar == 0) && all(diag(P_bar) == 0) 
        x_bar = zeros(15, 1);
        P_bar = 100 * I_15;
    end
    
    % State Decomposition
    epsi = x_bar(1:6);      % Wave states
    eta = x_bar(7:9);       % Position/heading
    b = x_bar(10:12);       % Bias
    nu = x_bar(13:15);      % Velocity
    
    u = nu(1);
    v = nu(2);
    r = nu(3);
    
    b1 = b(1);
    b2 = b(2);
    b3 = b(3);
    
    %% PREDICT STEP
    
    psi = eta(3);
    c_psi = cos(psi);
    s_psi = sin(psi);
    
    R_psi = [c_psi, -s_psi, 0;
             s_psi,  c_psi, 0;
             0,      0,     1];
    
    % Continuous-time dynamics f(x, tau)
    
    % Wave Dynamics (d_epsi)
    d_epsi = A_w * epsi;
    
    % Kinematics (d_eta)
    d_eta = R_psi * nu;
    
    % Bias Dynamics (d_b) - First-order decay
    d_b = -[b1/Tb1; b2/Tb2; b3/Tb3];
    
    % LF Dynamics (d_nu)
    % For diagonal mass and damping matrices
    d_nu = zeros(3,1);
    d_nu(1) = (1/m11) * (-d11*u + c_psi*b1 - s_psi*b2 + tau(1));
    d_nu(2) = (1/m22) * (-d22*v + s_psi*b1 + c_psi*b2 + tau(2));
    d_nu(3) = (1/m33) * (-d33*r + b3 + tau(3));
    
    % Full dynamics vector
    f = [d_epsi; d_eta; d_b; d_nu];
    
    % Predict state
    x_hat_minus = x_bar + Ts * f;
    
    %% Compute Jacobian A (15x15) - Continuous-time
    A = zeros(15, 15);
    
    % Row 1-3: d(d_epsi1-3)/dx (velocity part of wave model)
    A(1, 4) = 1;
    A(2, 5) = 1;
    A(3, 6) = 1;
    
    % Row 4-6: d(d_epsi4-6)/dx (acceleration part of wave model)
    A(4, 1) = -omega1^2;
    A(4, 4) = -2*omega1*zeta1;
    A(5, 2) = -omega2^2;
    A(5, 5) = -2*omega2*zeta2;
    A(6, 3) = -omega3^2;
    A(6, 6) = -2*omega3*zeta3;
    
    % Row 7-9: d(d_eta)/dx (kinematics)
    A(7, 9) = -v*c_psi - u*s_psi;  % d(dx)/d(psi)
    A(7, 13) = c_psi;               % d(dx)/d(u)
    A(7, 14) = -s_psi;              % d(dx)/d(v)
    
    A(8, 9) = u*c_psi - v*s_psi;   % d(dy)/d(psi)
    A(8, 13) = s_psi;               % d(dy)/d(u)
    A(8, 14) = c_psi;               % d(dy)/d(v)
    
    A(9, 15) = 1;                   % d(dpsi)/d(r)
    
    % Row 10-12: d(d_b)/dx (bias dynamics)
    A(10, 10) = -1/Tb1;
    A(11, 11) = -1/Tb2;
    A(12, 12) = -1/Tb3;
    
    % Row 13-15: d(d_nu)/dx (dynamics)
    A(13, 9) = -(b2*c_psi)/m11 - (b1*s_psi)/m11;  % d(du)/d(psi)
    A(13, 10) = c_psi/m11;                        % d(du)/d(b1)
    A(13, 11) = -s_psi/m11;                       % d(du)/d(b2)
    A(13, 13) = -d11/m11;                         % d(du)/d(u)
    
    A(14, 9) = (b1*c_psi)/m22 - (b2*s_psi)/m22;   % d(dv)/d(psi)
    A(14, 10) = s_psi/m22;                        % d(dv)/d(b1)
    A(14, 11) = c_psi/m22;                        % d(dv)/d(b2)
    A(14, 14) = -d22/m22;                         % d(dv)/d(v)
    
    A(15, 12) = 1/m33;                            % d(dr)/d(b3)
    A(15, 15) = -d33/m33;                         % d(dr)/d(r)
    
    % Discrete Jacobian
    F = I_15 + Ts * A;
    
    % Predict covariance
    P_minus = F * P_bar * F' + Q;
    
    %% UPDATE STEP
    
    % Measurement Jacobian H (3x15)
    % y = eta + C_w * epsi = [x; y; psi] + [epsi1; epsi2; epsi3]
    H = zeros(3, 15);
    H(1:3, 1:3) = I;      % d(y)/d(epsi_pos)
    H(1:3, 7:9) = I;      % d(y)/d(eta)
    
    % Predicted measurement
    epsi_pos_minus = x_hat_minus(1:3);
    eta_minus = x_hat_minus(7:9);
    y_hat_minus = eta_minus + epsi_pos_minus;
    
    % Innovation
    innovation = y - y_hat_minus;
    
    % Kalman Gain
    S = H * P_minus * H' + R;
    K = P_minus * H' / S;
    
    % Update state
    x_hat = x_hat_minus + K * innovation;
    
    % Update covariance (Joseph form)
    KH = K * H;
    P = (I_15 - KH) * P_minus * (I_15 - KH)' + K * R * K';
    
    %% Output
    x_bar_next = x_hat;  
    P_bar_next = P;
    
    eta_hat = x_hat(7:9);
    nu_hat = x_hat(13:15);
end

== matlab function part2/Observer/NED to BODY2 ==
  data: u input; m output; psi input
function m = fcn(u,psi)
    J = [cos(psi) -sin(psi) 0;
        sin(psi) cos(psi) 0;
        0 0 1];
    m = J'*u;

== matlab function part2/Observer/BODY to NED ==
  data: u input; m output; psi input
function m = fcn(u,psi)
    J = [cos(psi) -sin(psi) 0;
        sin(psi) cos(psi) 0;
        0 0 1];
    m = J*u;

== matlab function part2/Wind1/Wind Speed/MATLAB Function1 ==
  data: time input; U_gi output
function U_gi = fcn(time)
%Harris wind spectrum


Kappa = 0.0026; 
L = 1800; 
U_bar = 10;

f = linspace(0.001, 0.01, 1000);
df = f(2)-f(1);                       
phaseAngle = 2*pi*rand(1, 1000);

% Harris spectrum (Eq. 6.30)
f_tilde = L*f/U_bar;
S = (4*Kappa*L*U_bar) ./ ((2 + f_tilde.^2).^(5/6));

% Wind gust
U_gi = zeros(size(time));

for i=2:length(f)
    U_gi = U_gi + sqrt(2*S(i)*df)* cos(2*pi*time*f(i) + phaseAngle(i));
end

== matlab function part2/Thrust Allocation1/Normal/Thrust Allocation ==
  data: tau_D input; u output; alpha output; t_prev_new output; f0_new output; alpha_0_new output; s output; f0 input; alpha0 input; t input; t_prev input
function [u, alpha, t_prev_new, f0_new, alpha_0_new,s] = thrust_alloc(tau_D, f0, alpha0, t, t_prev)
% Inputs:
%   tau_D      : 6x1 desired generalized forces
%   f0         : 5x1 previous thrust commands (N)
%   alpha_0 : 5x1 previous azimuth angles (rad)
%   t          : current time (s)
%   t_prev     : previous time (s)
% Outputs:
%   u               : 5x1 updated thrust command (N)
%   s               : 3x1 slack variables
%   alpha           : 5x1 updated azimuth angles (rad)
%   t_prev_new      : for the next iteration
%   alpha_0_new  :  for the next iteration
%   f0_new  :  for the next iteration
u = zeros(5,1);
alpha = zeros(5,1);
s = zeros(3,1);
t_prev_new = 0;
f0_new = zeros(5,1);
alpha_0_new = zeros(5,1);

tau_3_D = [tau_D(1); tau_D(2); tau_D(6)];  % surge, sway, yaw
lx = [39.3, 36.5, 34.3, -28.5, -28.5];
ly = [0, 0, 0, 5, -5];

n_u = 5;
n_a = 5;
n_s = 3;
if isempty(f0) || isempty(alpha0) || isempty(t_prev)
    f0=zeros(n_u,1);
    alpha0=zeros(n_a,1);
    t_prev=0;
end
alpha0([1,3])=pi/2;

% --- time step
dt = t - t_prev;
if dt <= 0
    dt = 1e-3;
end

%  azimuth rate limit: 2 rpm -> rad/s ---
omega_max = 2 * 2*pi/60;   % rad/s = 0.20944
dalpha_max_step = omega_max * dt;

%  thruster absolute limits (N) and rise times (s) ---
f_max = [125; 150; 125; 300; 300] * 1000;   % N
f_min = 0; % Should be zero maybe? 

rise_time = [8; 8; 8; 10; 10];              % seconds for 0->100%
f_rate = f_max ./ rise_time;               % N/s per thruster
df_max = f_rate * dt;                 % max N change per iteration

%  delta bounds
lb_df = f_min - f0;
ub_df = f_max - f0;

ub_df = min(ub_df, df_max);         %Choose correct limit for delta f
lb_df = max(lb_df, -df_max);

%  delta alpha bounds
lb_da = -dalpha_max_step * ones(n_a,1);
ub_da =  dalpha_max_step * ones(n_a,1);
lb_da([1,3]) = 0;
ub_da([1,3]) = 0;

%  alpha bounds
alpha_min = -pi * ones(n_a,1);
alpha_max =  pi * ones(n_a,1);

lb_da = max(lb_da, alpha_min - alpha0);         %Choose correct limit for delta alpha
ub_da = min(ub_da, alpha_max - alpha0);

%  Slack bounds
lb_s = -Inf(n_s,1);
ub_s =  Inf(n_s,1);

lb = [lb_df; lb_da; lb_s];
ub = [ub_df; ub_da; ub_s];

%  Weight matrices 
P = 1e-8 * eye(n_u);       % weight on delta f (small)
Omega = 1e-8 * eye(n_a);   % weight on delta alpha (small)
Q = 1e6 * eye(n_s);        % heavy slack penalty

H = 2 * blkdiag(P, Omega, Q);       % quadprog expects 0.5 x' H x

%  Linear terms from quadratic expansions 
f_df = 2 * P * f0;                % from (f0 + df)' P (f0 + df)

%  Build T(alpha0) and dT/dalpha at alpha0 
T0 = T_alpha(alpha0, lx, ly);       % 3x5
dT = delT_delAlpha(alpha0, lx, ly); % cell 1x5 of 3x5 matrices

%  Compute M = [dT/dalpha]*f0  --> 3x5 matrix where col i = dT_i * f0 ---
dT_f0 = zeros(n_s, n_a);
for i = 1:n_a
    dT_f0(:,i) = dT{i} * f0;
end

% -avoid singular configurations 
sigma = 1.0; 
epsilon = 1e-12;
W = 1e-8 * eye(n_u);

g_det = gradient_g(T0, dT, W, sigma, epsilon); 

f_dalpha =  g_det;

% Full linear term for quadprog: f such that objective = 0.5 x'Hx + f'x
f = [f_df; f_dalpha; zeros(n_s,1)];

% Equality constraint: s + T0*Δf + dT_f0 * Δα = tau_3_D - T0*f0 
Aeq = [T0, dT_f0, eye(n_s)];   % 3 x (5 + 5 + 3)
beq = tau_3_D - T0 * f0;

%  Solve QP 
options = optimoptions('quadprog','Algorithm','active-set', 'Display','off','OptimalityTolerance',1e-9,'ConstraintTolerance',1e-9);

x0 = zeros(n_u + n_a + n_s, 1);
[x, exitflag] = quadprog(H, f, [], [], Aeq, beq, lb, ub, x0,options);

if isempty(x) || exitflag <= 0
    % Fallback: maintain previous commands, slack absorbs error
    delta_f = zeros(n_u, 1);
    delta_a = zeros(n_a, 1);
    s = beq;
else
    delta_f = x(1:n_u);
    delta_a = x(n_u+1:n_u+n_a);
    s = x(n_u+n_a+1:end);
end
%  outputs 
u = f0 + delta_f;
alpha = alpha0 + delta_a;


% Values for the next iteration
alpha_0_new = alpha;
f0_new = u;
t_prev_new = t;

% Ensure column vectors
u = u(:);
s = s(:);
alpha = alpha(:);

end

% Helper functions 

function Tmat = T_alpha(a, lx, ly)
    T1 = [0; 1; lx(1)];
    T2 = [cos(a(2)); sin(a(2)); lx(2)*sin(a(2))-ly(2)*cos(a(2))];
    T3 = [0; 1; lx(3)];
    T4 = [cos(a(4)); sin(a(4)); lx(4)*sin(a(4)) - ly(4)*cos(a(4))];
    T5 = [cos(a(5)); sin(a(5)); lx(5)*sin(a(5)) - ly(5)*cos(a(5))];
    Tmat = [T1 T2 T3 T4 T5];
end

function dT = delT_delAlpha(a, lx, ly)
 % returns 1x5 cell array where each cell is 3x5 dT/dalpha_i.

dT = cell(1,5);

% Thruster 1 (Tunnel)
dT{1} = zeros(3,5);

% Thruster 2 (Azimuth)
dT{2} = [
    0 -sin(a(2)) 0 0 0;
    0 cos(a(2)) 0 0 0;
    0 lx(2)*cos(a(2))+ly(2)*sin(a(2)) 0 0 0
];

% Thruster 3 (Tunnel)
dT{3} = zeros(3,5);

% Thruster 4 (Azimuth)
dT{4}=[
    0 0 0 -sin(a(4)) 0;
    0 0 0 cos(a(4)) 0;
    0 0 0 ( lx(4)*cos(a(4)) + ly(4)*sin(a(4))) 0
];

% Thruster 5 (Azimuth)
dT{5} = [
    0 0 0 0 -sin(a(5));
    0 0 0 0 cos(a(5));
    0 0 0 0 ( lx(5)*cos(a(5)) + ly(5)*sin(a(5)))
];


end

function del_g = gradient_g(Tm, dTcell, W, sigma, epsilon)
    % gradient of g(alpha) = sigma / (epsilon + det(X)) where X = T W^{-1} T'
    n_alpha = 5;
    del_g = zeros(n_alpha,1);
    Winv = diag(1 ./ diag(W)); % since W is diagonal
    X = Tm * Winv * Tm';
    detX = det(X);
    if detX <= 0
        return
    end
    Xinv = inv(X);
    for i = 1:n_alpha
        dT = dTcell{i};
        dX = dT * Winv * Tm' + Tm * Winv * dT';
        ddet = detX * trace(Xinv * dX);
        del_g(i) = -sigma * ddet / (epsilon + detX)^2;
    end
end

== matlab function part2/Current (North - East)1/MATLAB Function ==
  data: t input; Vc_NED output; Vc_mag input
function Vc_NED = LinearlyVaryingCurrent(t,Vc_mag)
theta = min(pi/2, (pi/2)*(t/300));  % angle in radians
Vc_NED = [Vc_mag*cos(theta) Vc_mag*sin(theta) 0];

== matlab function part2/Thrust Allocation1/Disabled Thrusters/Thrust Allocation ==
  data: tau_D input; u output; alpha output; t_prev_new output; f0_new output; alpha_0_new output; s output; f0 input; alpha0 input; t input; t_prev input
function [u, alpha, t_prev_new, f0_new, alpha_0_new,s] = thrust_alloc_disabled2and4(tau_D, f0, alpha0, t, t_prev)
% Inputs:
%   tau_D      : 6x1 desired generalized forces
%   f0         : 5x1 previous thrust commands (N)
%   alpha_0 : 5x1 previous azimuth angles (rad)
%   t          : current time (s)
%   t_prev     : previous time (s)
% Outputs:
%   u               : 5x1 updated thrust command (N)
%   s               : 3x1 slack variables
%   alpha           : 5x1 updated azimuth angles (rad)
%   t_prev_new      : for the next iteration
%   alpha_0_new  :  for the next iteration
%   f0_new  :  for the next iteration

u = zeros(5,1);
alpha = zeros(5,1);
s = zeros(3,1);
t_prev_new = 0;
f0_new = zeros(5,1);
alpha_0_new = zeros(5,1);

tau_3_D = [tau_D(1); tau_D(2); tau_D(6)];  % surge, sway, yaw
lx = [39.3, 36.5, 34.3, -28.5, -28.5];
ly = [0, 0, 0, 5, -5];

n_u = 5;
n_a = 5;
n_s = 3;
if isempty(f0) || isempty(alpha0) || isempty(t_prev)
    f0=zeros(n_u,1);
    alpha0=zeros(n_a,1);
    t_prev=0;
end
alpha0([1,3])=pi/2;

%  time step
dt = t - t_prev;
if dt <= 0
    dt = 1e-3;
end

%  azimuth rate limit: 2 rpm -> rad/s 
omega_max = 2 * 2*pi/60;   % rad/s = 0.20944
dalpha_max_step = omega_max * dt;

%  thruster absolute limits (N) and rise times (s) 
f_max = [125; 0; 125; 0; 300] * 1000;   % N
f_min = -f_max;

rise_time = [8; 8; 8; 10; 10];         % seconds for 0->100%
f_rate = f_max ./ rise_time;               % N/s per thruster
df_max = f_rate * dt;                 % max N change per iteration

%  delta bounds for thrust 
lb_df = f_min - f0;
ub_df = f_max - f0;

ub_df = min(ub_df, df_max);         %Choose correct limit for delta f
lb_df = max(lb_df, -df_max);

%  delta alpha bounds
lb_da = -dalpha_max_step * ones(n_a,1);
ub_da =  dalpha_max_step * ones(n_a,1);
lb_da([1,3]) = 0;
ub_da([1,3]) = 0;

%  alpha bounds
alpha_min = -pi * ones(n_a,1);
alpha_max =  pi * ones(n_a,1);

lb_da = max(lb_da, alpha_min - alpha0);         %Choose correct limit for delta alpha
ub_da = min(ub_da, alpha_max - alpha0);

%  Slack bounds 
lb_s = -Inf(n_s,1);
ub_s =  Inf(n_s,1);

lb = [lb_df; lb_da; lb_s];
ub = [ub_df; ub_da; ub_s];

%  Weight matrices 
P = (1e-8 * eye(n_u));       % weight on delta f (small)
Omega = (1e-8 * eye(n_a));   % weight on delta alpha (small)
Q = (1e6 * eye(n_s));        % heavy slack penalty

H = 2 * blkdiag(P, Omega, Q);       % quadprog expects 0.5 x' H x

%  Linear terms from quadratic expansions 
f_df = 2 * P * f0;                % from (f0 + df)' P (f0 + df)

%  Build T(alpha0) and dT/dalpha at alpha0 
T0 = T_alpha(alpha0, lx, ly);       % 3x5
dT = delT_delAlpha(alpha0, lx, ly); % cell 1x5 of 3x5 matrices

%  Compute M = [dT/dalpha]*f0  --> 3x5 matrix where col i = dT_i * f0 
dT_f0 = zeros(n_s, n_a);
for i = 1:n_a
    dT_f0(:,i) = dT{i} * f0;
end

%  avoid singular configurations 
sigma = 1.0;
epsilon = 1e-12;
W = 1e-8 * eye(n_u);

g_det = gradient_g(T0, dT, W, sigma, epsilon); 

f_dalpha =  g_det;

% Full linear term for quadprog: f such that objective = 0.5 x'Hx + f'x
f = [f_df; f_dalpha; zeros(n_s,1)];

%  Equality constraint: s + T0*Δf + dT_f0 * Δα = tau_3_D - T0*f0 
Aeq = [T0, dT_f0, eye(n_s)];   % 3 x (5 + 5 + 3)
beq = tau_3_D - T0 * f0;

%  Solve QP 

options = optimoptions('quadprog','Algorithm','active-set', 'Display','off','OptimalityTolerance',1e-9,'ConstraintTolerance',1e-9);

x0 = zeros(n_u + n_a + n_s, 1);
[x, exitflag] = quadprog(H, f, [], [], Aeq, beq, lb, ub, x0,options);
% Handle solver failure
if isempty(x) || exitflag <= 0
    % Fallback: maintain previous thrust, slack absorbs error
    delta_f = zeros(n_u, 1);
    delta_a = zeros(n_a, 1);
    s = beq;
else
    delta_f = x(1:n_u);
    delta_a = x(n_u+1:n_u+n_a);
    s = x(n_u+n_a+1:end);
end

% \ outputs
u = f0 + delta_f;
alpha = alpha0 + delta_a;


% Values for the next iteration
alpha_0_new = alpha;
f0_new = u;
t_prev_new = t;

% Ensure column vectors
u = u(:);
s = s(:);
alpha = alpha(:);

end

% Helper functions 

function Tmat = T_alpha(a, lx, ly)
    T1 = [0; 1; lx(1)];
    T2 = zeros(3, 1);  % Disabled thruster 2
    T3 = [0; 1; lx(3)];
    T4 = zeros(3, 1);  % Disabled thruster 4
    T5 = [cos(a(5)); sin(a(5)); lx(5)*sin(a(5)) - ly(5)*cos(a(5))];
    Tmat = [T1 T2 T3 T4 T5];
end

function dT = delT_delAlpha(a, lx, ly)
 % returns 1x5 cell array where each cell is 3x5 dT/dalpha_i.

dT = cell(1,5);

% Thruster 1 (Tunnel)
dT{1} = zeros(3,5);

% Thruster 2 (Azimuth)
dT{2} =  zeros(3,5);

% Thruster 3 (Tunnel)
dT{3} = zeros(3,5);

% Thruster 4 (Azimuth)
dT{4}=zeros(3,5);

% Thruster 5 (Azimuth)
dT{5} = [
    0 0 0 0 -sin(a(5));
    0 0 0 0 cos(a(5));
    0 0 0 0 ( lx(5)*cos(a(5)) + ly(5)*sin(a(5)))
];


end

function del_g = gradient_g(Tm, dTcell, W, sigma, epsilon)
    % gradient of g(alpha) = sigma / (epsilon + det(X)) where X = T W^{-1} T'
    n_alpha = 5;
    del_g = zeros(n_alpha,1);
    Winv = diag(1 ./ diag(W)); % since W is diagonal
    X = Tm * Winv * Tm';
    detX = det(X);
    if detX <= 0
        return
    end
    Xinv = inv(X);
    for i = 1:n_alpha
        dT = dTcell{i};
        dX = dT * Winv * Tm' + Tm * Winv * dT';
        ddet = detX * trace(Xinv * dX);
        del_g(i) = -sigma * ddet / (epsilon + detX)^2;
    end
end

== matlab function part2/Thruster Dynamics/MATLAB Function ==
  data: alpha_actual input; thrust_actual input; actual_tau output; PosX input; PosY input
function actual_tau   = fcn(alpha_actual,thrust_actual,PosX,PosY)

    Alpha_surge =[cos(alpha_actual(1)) cos(alpha_actual(2)) cos(alpha_actual(3)) cos(alpha_actual(4)) cos(alpha_actual(5))];  
    Alpha_sway = [sin(alpha_actual(1)) sin(alpha_actual(2)) sin(alpha_actual(3)) sin(alpha_actual(4)) sin(alpha_actual(5))];
    Alpha_yaw = [sin(alpha_actual(1))*PosX(1)-cos(alpha_actual(1))*PosY(1) sin(alpha_actual(2))*PosX(2)-cos(alpha_actual(2))*PosY(2) ...
                 sin(alpha_actual(3))*PosX(3)-cos(alpha_actual(3))*PosY(3) sin(alpha_actual(4))*PosX(4)-cos(alpha_actual(4))*PosY(4) ...
                 sin(alpha_actual(5))*PosX(5)-cos(alpha_actual(5))*PosY(5)];

    actual_tau = [Alpha_surge; Alpha_sway; Alpha_yaw]*thrust_actual;
end

== matlab function part2/Current (North - East)1/MATLAB Function1 ==
  data: u1 input; y output; u2 input; u3 input; flag input
function y = fcn(u1, u2, u3, flag)

y = zeros(1,3);
switch flag
    case 1
        y(1:3) = u1;
    case 2
        y(1:3) = u2;
    case 3
        y(1:3) = u3;
    otherwise
        y(1:3) = u1;
end

== matlab function part2/Observer/NED to BODY ==
  data: u input; m output; psi input
function m = fcn(u,psi)
    J = [cos(psi) -sin(psi) 0;
        sin(psi) cos(psi) 0;
        0 0 1];
    m = J'*u;

== matlab function part2/DP Controller1/MATLAB Function ==
  data: u input; y output; eta input
function y = Rz_psi_T(u, eta)
y = zeros(3,1);

psi = eta(3);

c = cos(psi); s = sin(psi);

R = [c -s  0;
     s  c  0;
     0  0  1];

y = R'*u;

== matlab function part2/DP Controller1/MATLAB Function1 ==
  data: u input; y output; eta input
function y = Rz_psi(u, eta)
y = zeros(3,1);

psi = eta(3);

c = cos(psi); s = sin(psi);

R = [c -s  0;
     s  c  0;
     0  0  1];

y = R*u;
